simulink model "adaptiveIPDComboSim"  (R2016b)
settings: Solver=VariableStepAuto  StartTime=0.0  StopTime=500  RelTol=1e-3
undefined symbols (not defined in the file or in its folder): tf1
settings Model: Creator=julianleland  LastModifiedBy=julianleland

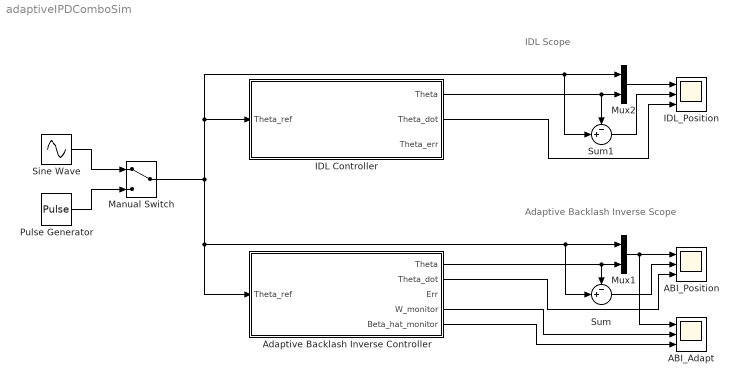
== system adaptiveIPDComboSim ==
  note: Adaptive Backlash Inverse Scope
  note: IDL Scope
  ABI_Adapt : Scope  NumInputPorts=3
  ABI_Position : Scope  NumInputPorts=3
  Adaptive Backlash Inverse Controller : Subsystem
  IDL Controller : Subsystem
  IDL_Position : Scope  NumInputPorts=3
  Manual Switch : ManualSwitch
  Mux1 : Mux  Inputs=2
  Mux2 : Mux  Inputs=2
  Pulse Generator : DiscretePulseGenerator  PulseType=Time based  Period=50  PulseWidth=50  PhaseDelay=0.5
  Sine Wave : Sin  Amplitude=2  SampleTime=0
  Sum : Sum  Inputs=-+|
  Sum1 : Sum  Inputs=-+|
  wires:
  IDL Controller/1(Theta) -> Sum1/1, Mux2/2
  Mux1/1 -> ABI_Adapt/1, ABI_Position/1
  Sum/1 -> ABI_Position/2
  Adaptive Backlash Inverse Controller/1(Theta) -> Sum/1, Mux1/2
  Mux2/1 -> IDL_Position/1
  Sum1/1 -> IDL_Position/2
  IDL Controller/2(Theta_dot) -> IDL_Position/3
  Adaptive Backlash Inverse Controller/2(Theta_dot) -> ABI_Position/3
  Manual Switch/1 -> Sum/2, Mux1/1, Adaptive Backlash Inverse Controller/1(Theta_ref), IDL Controller/1(Theta_ref), Sum1/2, Mux2/1
  Sine Wave/1 -> Manual Switch/1
  Pulse Generator/1 -> Manual Switch/2
  Adaptive Backlash Inverse Controller/5(Beta_hat_monitor) -> ABI_Adapt/3
  Adaptive Backlash Inverse Controller/4(W_monitor) -> ABI_Adapt/2

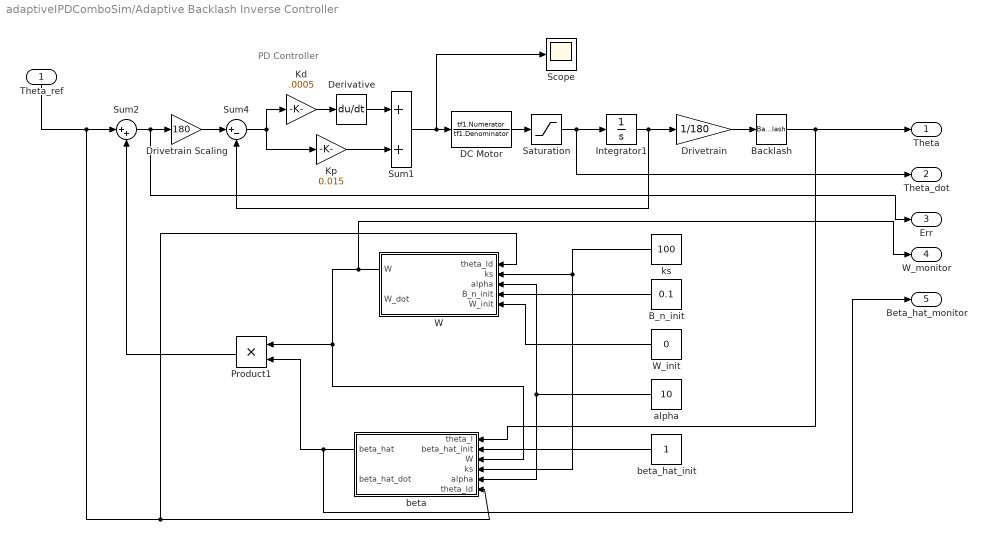
== system adaptiveIPDComboSim/Adaptive Backlash Inverse Controller ==
  note: PD Controller
  Theta_ref : Inport
  B_n_init : Constant  Value=0.1
  Backlash : Backlash  BacklashWidth=0.25
  DC Motor : TransferFcn  Numerator=tf1.Numerator  Denominator=tf1.Denominator
  Derivative : Derivative
  Drivetrain : Gain  Gain=1/180
  Drivetrain Scaling : Gain  Gain=180
  Integrator1 : Integrator
  Kd : Gain  Gain=.0005
  Kp : Gain  Gain=0.015
  Product1 : Product
  Saturation : Saturate  UpperLimit=460  LowerLimit=-460
  Scope : Scope
  Sum1 : Sum
  Sum2 : Sum  Inputs=|++
  Sum4 : Sum  Inputs=|+-
  W : Subsystem
  W_init : Constant  Value=0
  alpha : Constant  Value=10
  beta : Subsystem
  beta_hat_init : Constant
  ks : Constant  Value=100
  Theta : Outport
  Theta_dot : Outport  Port=2
  Err : Outport  Port=3
  W_monitor : Outport  Port=4
  Beta_hat_monitor : Outport  Port=5
  wires:
  Sum2/1 -> Err/1, Drivetrain Scaling/1
  Theta_ref/1 -> Sum2/1, W/1(theta_ld), beta/6(theta_ld)
  Integrator1/1 -> Sum4/2, Drivetrain/1
  beta_hat_init/1 -> beta/2(beta_hat_init)
  beta/1(beta_hat) -> Beta_hat_monitor/1, Product1/2
  alpha/1 -> beta/5(alpha), W/3(alpha)
  Kp/1 -> Sum1/2
  Kd/1 -> Derivative/1
  ks/1 -> beta/4(ks), W/2(ks)
  Sum1/1 -> Scope/1, DC Motor/1
  W/1(W) -> W_monitor/1, beta/3(W), Product1/1
  B_n_init/1 -> W/4(B_n_init)
  Saturation/1 -> Theta_dot/1, Integrator1/1
  W_init/1 -> W/5(W_init)
  Drivetrain/1 -> Backlash/1
  Sum4/1 -> Kd/1, Kp/1
  Derivative/1 -> Sum1/1
  Drivetrain Scaling/1 -> Sum4/1
  Product1/1 -> Sum2/2
  Backlash/1 -> Theta/1, beta/1(theta_l)
  DC Motor/1 -> Saturation/1

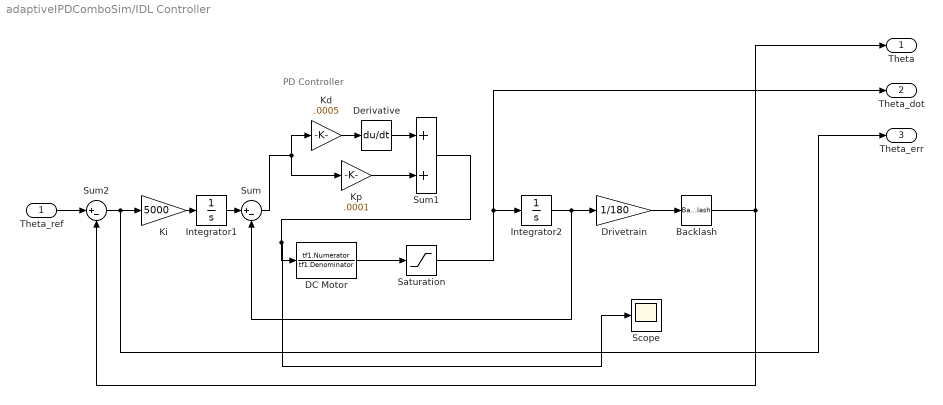
== system adaptiveIPDComboSim/IDL Controller ==
  note: PD Controller
  Theta_ref : Inport
  Backlash : Backlash  BacklashWidth=0.25
  DC Motor : TransferFcn  Numerator=tf1.Numerator  Denominator=tf1.Denominator
  Derivative : Derivative
  Drivetrain : Gain  Gain=1/180
  Integrator1 : Integrator  LimitOutput=on  UpperSaturationLimit=500  LowerSaturationLimit=-500
  Integrator2 : Integrator
  Kd : Gain  Gain=.0005
  Ki : Gain  Gain=5000
  Kp : Gain  Gain=.0001
  Saturation : Saturate  UpperLimit=460  LowerLimit=-460
  Scope : Scope
  Sum : Sum  Inputs=|+-
  Sum1 : Sum
  Sum2 : Sum  Inputs=|+-
  Theta : Outport
  Theta_dot : Outport  Port=2
  Theta_err : Outport  Port=3
  wires:
  Integrator1/1 -> Sum/1
  Theta_ref/1 -> Sum2/1
  Saturation/1 -> Theta_dot/1, Integrator2/1
  Backlash/1 -> Theta/1, Sum2/2
  Kd/1 -> Derivative/1
  DC Motor/1 -> Saturation/1
  Sum/1 -> Kp/1, Kd/1
  Derivative/1 -> Sum1/1
  Kp/1 -> Sum1/2
  Integrator2/1 -> Sum/2, Drivetrain/1
  Drivetrain/1 -> Backlash/1
  Ki/1 -> Integrator1/1
  Sum2/1 -> Theta_err/1, Ki/1
  Sum1/1 -> Scope/1, DC Motor/1

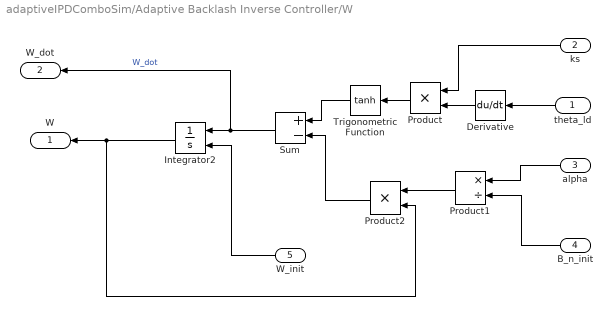
== system adaptiveIPDComboSim/Adaptive Backlash Inverse Controller/W ==
  theta_ld : Inport
  ks : Inport  Port=2
  alpha : Inport  Port=3
  B_n_init : Inport  Port=4
  W_init : Inport  Port=5
  Derivative : Derivative
  Integrator2 : Integrator  InitialConditionSource=external
  Product : Product
  Product1 : Product  Inputs=*/
  Product2 : Product
  Sum : Sum  Inputs=+-
  Trigonometric Function : Trigonometry  Operator=tanh
  W : Outport
  W_dot : Outport  Port=2
  wires:
  Product2/1 -> Sum/2
  W_init/1 -> Integrator2/2
  Sum/1 -> Integrator2/1, W_dot/1  "W_dot"
  Trigonometric Function/1 -> Sum/1
  theta_ld/1 -> Derivative/1
  Product/1 -> Trigonometric Function/1
  Product1/1 -> Product2/1
  B_n_init/1 -> Product1/2
  alpha/1 -> Product1/1
  ks/1 -> Product/1
  Derivative/1 -> Product/2
  Integrator2/1 -> W/1, Product2/2

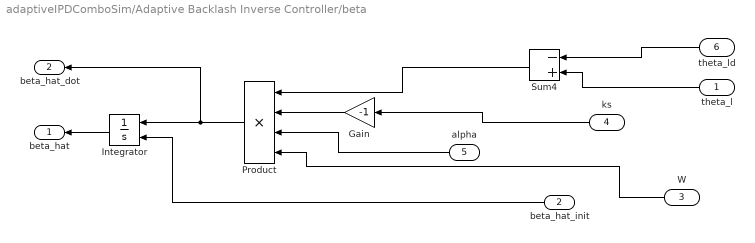
== system adaptiveIPDComboSim/Adaptive Backlash Inverse Controller/beta ==
  theta_l : Inport
  beta_hat_init : Inport  Port=2
  W : Inport  Port=3
  ks : Inport  Port=4
  alpha : Inport  Port=5
  theta_ld : Inport  Port=6
  Gain : Gain  Gain=-1
  Integrator : Integrator  InitialConditionSource=external
  Product : Product  Inputs=****
  Sum4 : Sum  Inputs=-+
  beta_hat : Outport
  beta_hat_dot : Outport  Port=2
  wires:
  beta_hat_init/1 -> Integrator/2
  Integrator/1 -> beta_hat/1
  ks/1 -> Gain/1
  theta_ld/1 -> Sum4/1
  theta_l/1 -> Sum4/2
  alpha/1 -> Product/3
  W/1 -> Product/4
  Gain/1 -> Product/2
  Product/1 -> beta_hat_dot/1, Integrator/1
  Sum4/1 -> Product/1
